simulink model "SF044A_HowDetn"  (R2013b)
settings: Solver=FixedStepDiscrete  SolverMode=SingleTasking  StartTime=0.0  StopTime=1  FixedStep=0.002  RelTol=1e-3
values from neighbouring files (symbols this model uses):
  ABSLTHIFRQTQHILIM_HWNWTMTR_F32 = DataDict.Constant    [SF044A_HowDetn_DataDict.m]
  ABSLTHIFRQTQLOLIM_HWNWTMTR_F32 = DataDict.Constant    [SF044A_HowDetn_DataDict.m]
  ARCHGLBPRM_2MILLISEC_SEC_F32 = DataDict.Constant    [SF044A_HowDetn_DataDict.m]
  HOWDETNESTIMNLIM_ULS_F32 = DataDict.Constant    [SF044A_HowDetn_DataDict.m]
  HOWDETNESTIMNTHD_ULS_F32 = DataDict.Constant    [SF044A_HowDetn_DataDict.m]
  HowDetnHiFrqGainY = DataDict.Calibration    [SF044A_HowDetn_DataDict.m]
  HowDetnMinVehSpd = DataDict.Calibration    [SF044A_HowDetn_DataDict.m]
  HowDetnPercOfPrevHowEstim = DataDict.Calibration    [SF044A_HowDetn_DataDict.m]
  HowDetnSlewRate = DataDict.Calibration    [SF044A_HowDetn_DataDict.m]
  HowDetnVehSpd = DataDict.Calibration    [SF044A_HowDetn_DataDict.m]
libraries: Fil x14, FloatToFixd x6, NxtrLim x5, FixdToFloat x3, BilnrIntrpnMplX x2, NxtrAbslt x2, simulink x2, LnrIntrpn x1, LnrIntrpnDyn x1
(part 1 of 2)
settings Model: Creator=xzqqlw  LastModifiedBy=XZB1DB
settings SolverCC: AutoInsertRateTranBlk=on  InsertRTBMode=Always
settings DataIOCC: LimitDataPoints=off  SaveFormat=Structure  ReturnWorkspaceOutputs=on
settings OptimizationCC: BlockReduction=off  InlineParams=on  ZeroExternalMemoryAtStartup=off  ZeroInternalMemoryAtStartup=off  OptimizeModelRefInitCode=on  LifeSpan=1
settings DebuggingCC: SignalInfNanChecking=error  SignalRangeChecking=warning  UnderspecifiedInitializationDetection=Simplified  SolverPrmCheckMsg=error  InheritedTsInSrcMsg=error  DiscreteInheritContinuousMsg=error  SingleTaskRateTransMsg=error  TasksWithSamePriorityMsg=error  SigSpecEnsureSampleTimeMsg=error  CheckMatrixSingularityMsg=error  ParameterUnderflowMsg=error  ParameterPrecisionLossMsg=error  ParameterTunabilityLossMsg=error  FixptConstUnderflowMsg=warning  FixptConstOverflowMsg=warning  VectorMatrixConversionMsg=error  SignalLabelMismatchMsg=error  UnconnectedInputMsg=error  UnconnectedOutputMsg=error  UnconnectedLineMsg=error  SFcnCompatibilityMsg=error  UniqueDataStoreMsg=warning  BusObjectLabelMismatch=error  RootOutportRequireBusObject=error  AssertControl=DisableAll  ModelReferenceIOMsg=error  ModelReferenceVersionMismatchMessage=warning  ModelReferenceIOMismatchMessage=error  ModelReferenceCSMismatchMessage=warning  ModelReferenceDataLoggingMessage=error  StateNameClashWarn=warning  StrictBusMsg=ErrorOnBusTreatedAsVector  NonBusSignalsTreatedAsBus=error  SFUnexpectedBacktrackingDiag=error  SFInvalidInputDataAccessInChartInitDiag=error  SFNoUnconditionalDefaultTransitionDiag=error  SFTransitionOutsideNaturalParentDiag=error  SFUnconditionalTransitionShadowingDiag=error  SFUndirectedBroadcastEventsDiag=error
settings ModelReferenceCC: ModelReferenceNumInstancesAllowed=Single
settings RTWCC: SystemTargetFile=autosar.tlc  GenCodeOnly=on  TemplateMakefile=ert_default_tmf  Description=AUTOSAR  GenerateReport=on  ProcessScript=autosar_make_rtw_hook  LaunchReport=on
settings CodeAppCC: GenerateComments=off  IgnoreCustomStorageClasses=off  CustomSymbolStrType=$N$R$M  CustomSymbolStrBlkIO=$N$M  SimulinkBlockComments=off
settings STFCustomTargetCC: ParMdlRefBuildCompliant=on  CompOptLevelCompliant=on  IncludeMdlTerminateFcn=off  CombineOutputUpdateFcns=on  SuppressErrorStatus=on  ERTFirstTimeCompliant=on  ERTCustomFileBanners=on  SupportNonFinite=off  SupportComplex=off  SupportContinuousTime=off  SupportNonInlinedSFcns=off  MATLABClassNameForMDSCustomization=Simulink.SoftwareTarget.ERTCustomization  AutosarCompliant=on  GRTInterface=off  SystemTargetFile=autosar.tlc
settings ERTTargetCC: CodeReplacementLibrary=ANSI_C  ConcurrentExecutionCompliant=off  IncludeMdlTerminateFcn=off  SuppressErrorStatus=on  SupportNonFinite=off  SupportComplex=off  ModelStepFunctionPrototypeControlCompliant=off  CPPClassGenCompliant=off  AutosarCompliant=on  InlinedParameterPlacement=NonHierarchical  ERTCustomFileTemplate=example_file_process.tlc  EnableUserReplacementTypes=on

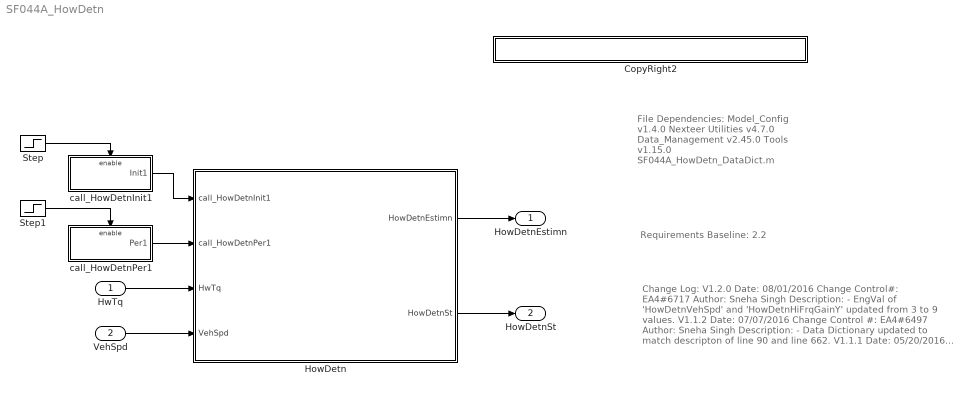
== system SF044A_HowDetn ==
  note: Change Log:
      |
      | V1.2.0
      | Date: 08/01/2016
      | Change Control#: EA4#6717
      | Author: Sneha Singh
      | Description:
      | - EngVal of 'HowDetnVehSpd' and 'HowDetnHiFrqGainY'
      | updated from 3 to 9 values.
      |
      | V1.1.2
      | Date: 07/07/2016
      | Change Control #: EA4#6497
      | Author: Sneha Singh
      | Description:
      | - Data Dictionary updated to match descripton
      | of line 90 and line 662.
      |
      | V1.1.1
      | Date: 05/20/2016
      | Change Control #: EA4#5844
      | Author: Sneha Singh
      | Description:
      | - Model traceability performed in DOORS.
      |
      | V 1.1.0
      | Date : 2/9/2016
      | Change Control #: EA4#2979
      | Author : Sudeep Shankar
      | Description:
      | - Limit block added to outputs 'HowDetnEstimn'.
      | and 'HowDetnSt'
      | - Updated DD to include 4 new constants
      |
      | V 1.0.0
      | Date: 1/14/2016
      | Change Control #: EA4#2979
      | Author: Sudeep Shankar
      | Description:
      | - Initial Release Based on EA3 V 1.0.0
  note: File Dependencies:
      |
      | Model_Config v1.4.0
      | Nexteer Utilities v4.7.0
      | Data_Management v2.45.0
      | Tools v1.15.0
      | SF044A_HowDetn_DataDict.m
  note: Requirements Baseline: 2.2
  HwTq : Inport  RequirementInfo={'linktype_rmi_doors' '0000baa4 (/E-STEER Core/SubSystem Specifications/Application Functions/SF044A HOW)' '#SF044A_67' 'true' 'REQ:SF044A_67' '' } %GIDa_72f413cc_dc3e_4eb0_8a2d_65e9c1fff85e
  VehSpd : Inport  RequirementInfo={'linktype_rmi_doors' '0000baa4 (/E-STEER Core/SubSystem Specifications/Application Functions/SF044A HOW)' '#SF044A_68' 'true' 'REQ:SF044A_68' '' } %GIDa_cc4347af_bdaf_4f30_b9d2_4f20a9b04acc  Port=2
  CopyRight2 : Subsystem  Description=|  mask(Copyright Information){none=on}
      | Copyright info block.                                               
      |                                                                     
      | Place copyright information at the top of every subsystem in design.
      mask prompts: none "No parameters"
      mask help: Place copyright information at the top of every subsystem in design.
      mask Display:
      | NxtrConf = 'Nexteer Confidential';
      | 
      | sys = bdroot; %handle for the current model ("system")
      | first = get_param(sys,'Created');
      | if(isempty(first))
      |     first = datestr(now,'yyyy');
      | else
      |     first = first(end-3:end);  %year is last four digits
      | end
      | 
      | last = get_param(sys,'LastModifiedDate');
      | if isempty(last)
      |     last = datestr(now,'yyyy');
      | else
      |     last = last(end-3:end);
      | end
      | 
      | if strcmp(first,last)
      |     fprintf('%s -- Copyright %s Nexteer',NxtrConf,first)
      | else
      |     fprintf('%s -- %s%s- %s Nexteer',NxtrConf,char(169),first,last)
      | end
  HowDetn : Subsystem
  Step : Step  Time=.001  Before=1  After=0  SampleTime=0
  Step1 : Step  Time=.001  SampleTime=0
  call_HowDetnInit1 : Subsystem  TreatAsAtomicUnit=on
  call_HowDetnPer1 : Subsystem  TreatAsAtomicUnit=on
  HowDetnEstimn : Outport  RequirementInfo={'linktype_rmi_doors' '0000baa4 (/E-STEER Core/SubSystem Specifications/Application Functions/SF044A HOW)' '#SF044A_69' 'true' 'REQ:SF044A_69' '' } %GIDa_72335151_86e3_4c12_b306_092b88286120
  HowDetnSt : Outport  RequirementInfo={'linktype_rmi_doors' '0000baa4 (/E-STEER Core/SubSystem Specifications/Application Functions/SF044A HOW)' '#SF044A_70' 'true' 'REQ:SF044A_70' '' } %GIDa_5536db44_27aa_4fe7_bd69_6a82a7bbddee  Port=2
  wires:
  HwTq/1 -> HowDetn/3(HwTq)
  HowDetn/1(HowDetnEstimn) -> HowDetnEstimn/1
  VehSpd/1 -> HowDetn/4(VehSpd)
  call_HowDetnPer1/1(Per1) -> HowDetn/2(call_HowDetnPer1)
  Step/1 -> call_HowDetnInit1/Enable
  call_HowDetnInit1/1(Init1) -> HowDetn/1(call_HowDetnInit1)
  Step1/1 -> call_HowDetnPer1/Enable
  HowDetn/2(HowDetnSt) -> HowDetnSt/1

== system SF044A_HowDetn/CopyRight2 ==

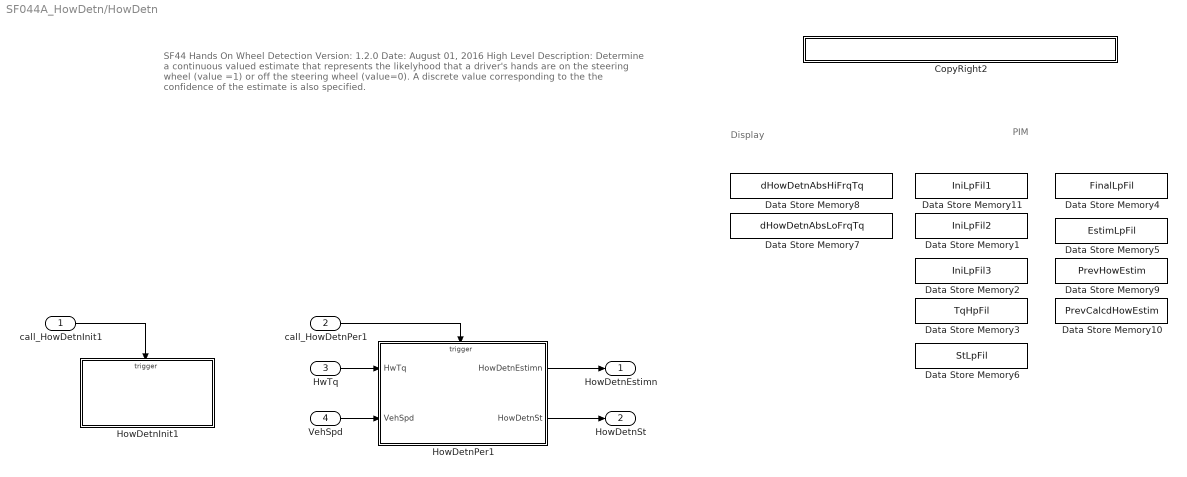
== system SF044A_HowDetn/HowDetn ==
  note: SF44 Hands On Wheel Detection
      |          Version:  1.2.0          Date: August 01, 2016
      |
      | High Level Description:
      | Determine a continuous valued estimate that represents the likelyhood that a driver's hands are
      | on the steering wheel (value =1) or off the steering wheel (value=0).  A discrete value corresponding
      | to the the confidence of the estimate is also specified.
  note: Display
  note: PIM
  call_HowDetnInit1 : Inport
  call_HowDetnPer1 : Inport  Port=2
  HwTq : Inport  Port=3
  VehSpd : Inport  Port=4
  CopyRight2 : Subsystem  Description=|  mask(Copyright Information){none=on}
      | Copyright info block.                                               
      |                                                                     
      | Place copyright information at the top of every subsystem in design.
      mask prompts: none "No parameters"
      mask help: Place copyright information at the top of every subsystem in design.
      mask Display:
      | NxtrConf = 'Nexteer Confidential';
      | 
      | sys = bdroot; %handle for the current model ("system")
      | first = get_param(sys,'Created');
      | first = first(end-3:end);  %year is last four digits
      | 
      | last = get_param(sys,'LastModifiedDate');
      | if isempty(last)
      |     last = datestr(now,'yyyy');
      | else
      |     last = last(end-3:end);
      | end
      | 
      | if strcmp(first,last)
      |     fprintf('%s -- Copyright %s Nexteer',NxtrConf,first)
      | else
      |     fprintf('%s -- %s%s- %s Nexteer',NxtrConf,char(169),first,last)
      | end
  Data Store Memory1 : DataStoreMemory  DataStoreName=IniLpFil2  InitialValue=struct( 'FilSt' , single(0) , 'FilGain', single(0) )  OutDataTypeStr=Bus: FilLpRec1  StateMustResolveToSignalObject=on
  Data Store Memory10 : DataStoreMemory  DataStoreName=PrevCalcdHowEstim  StateMustResolveToSignalObject=on
  Data Store Memory11 : DataStoreMemory  DataStoreName=IniLpFil1  InitialValue=struct( 'FilSt' , single(0) , 'FilGain', single(0) )  OutDataTypeStr=Bus: FilLpRec1  StateMustResolveToSignalObject=on
  Data Store Memory2 : DataStoreMemory  DataStoreName=IniLpFil3  InitialValue=struct( 'FilSt' , single(0) , 'FilGain', single(0) )  OutDataTypeStr=Bus: FilLpRec1  StateMustResolveToSignalObject=on
  Data Store Memory3 : DataStoreMemory  DataStoreName=TqHpFil  InitialValue=struct( 'FilLpRec' , struct( 'FilSt' , single(0) , 'FilGain', single(0) ) , 'CorrnFac', single(0) )  OutDataTypeStr=Bus: FilHpRec1  StateMustResolveToSignalObject=on
  Data Store Memory4 : DataStoreMemory  DataStoreName=FinalLpFil  InitialValue=struct( 'FilSt' , single(0) , 'FilGain', single(0) )  OutDataTypeStr=Bus: FilLpRec1  StateMustResolveToSignalObject=on
  Data Store Memory5 : DataStoreMemory  DataStoreName=EstimLpFil  InitialValue=struct( 'FilSt' , single(0) , 'FilGain', single(0) )  OutDataTypeStr=Bus: FilLpRec1  StateMustResolveToSignalObject=on
  Data Store Memory6 : DataStoreMemory  DataStoreName=StLpFil  InitialValue=[]  OutDataTypeStr=Bus: FilLpRec1  StateMustResolveToSignalObject=on
  Data Store Memory7 : DataStoreMemory  DataStoreName=dHowDetnAbsLoFrqTq  StateMustResolveToSignalObject=on
  Data Store Memory8 : DataStoreMemory  DataStoreName=dHowDetnAbsHiFrqTq  StateMustResolveToSignalObject=on
  Data Store Memory9 : DataStoreMemory  DataStoreName=PrevHowEstim  StateMustResolveToSignalObject=on
  HowDetnInit1 : Subsystem
  HowDetnPer1 : Subsystem  RequirementInfo={} %GIDa_2a73c725_3b58_4254_b96a_f86bf171ea48
  HowDetnEstimn : Outport
  HowDetnSt : Outport  Port=2
  wires:
  HwTq/1 -> HowDetnPer1/1(HwTq)
  call_HowDetnPer1/1 -> HowDetnPer1/Trigger
  call_HowDetnInit1/1 -> HowDetnInit1/Trigger
  HowDetnPer1/1(HowDetnEstimn) -> HowDetnEstimn/1
  HowDetnPer1/2(HowDetnSt) -> HowDetnSt/1
  VehSpd/1 -> HowDetnPer1/2(VehSpd)

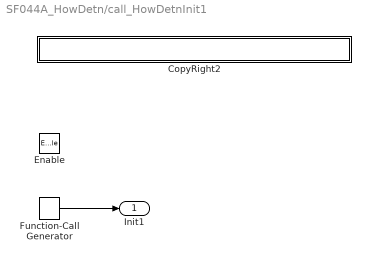
== system SF044A_HowDetn/call_HowDetnInit1 ==
  Enable : EnablePort
  CopyRight2 : Subsystem  Description=|  mask(Copyright Information){none=on}
      | Copyright info block.                                               
      |                                                                     
      | Place copyright information at the top of every subsystem in design.
      mask prompts: none "No parameters"
      mask help: Place copyright information at the top of every subsystem in design.
      mask Display:
      | NxtrConf = 'Nexteer Confidential';
      | 
      | sys = bdroot; %handle for the current model ("system")
      | first = get_param(sys,'Created');
      | if(isempty(first))
      |     first = datestr(now,'yyyy');
      | else
      |     first = first(end-3:end);  %year is last four digits
      | end
      | 
      | last = get_param(sys,'LastModifiedDate');
      | if isempty(last)
      |     last = datestr(now,'yyyy');
      | else
      |     last = last(end-3:end);
      | end
      | 
      | if strcmp(first,last)
      |     fprintf('%s -- Copyright %s Nexteer',NxtrConf,first)
      | else
      |     fprintf('%s -- %s%s- %s Nexteer',NxtrConf,char(169),first,last)
      | end
  Function-Call Generator : simulink/Ports & Subsystems/Function-Call Generator  sample_time=.004  numberOfIterations=1
  Init1 : Outport
  wires:
  Function-Call Generator/1 -> Init1/1

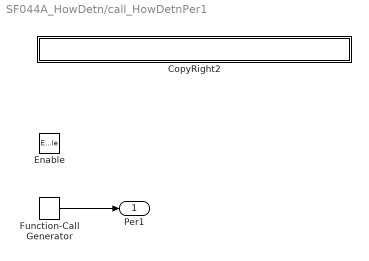
== system SF044A_HowDetn/call_HowDetnPer1 ==
  Enable : EnablePort
  CopyRight2 : Subsystem  Description=|  mask(Copyright Information){none=on}
      | Copyright info block.                                               
      |                                                                     
      | Place copyright information at the top of every subsystem in design.
      mask prompts: none "No parameters"
      mask help: Place copyright information at the top of every subsystem in design.
      mask Display:
      | NxtrConf = 'Nexteer Confidential';
      | 
      | sys = bdroot; %handle for the current model ("system")
      | first = get_param(sys,'Created');
      | if(isempty(first))
      |     first = datestr(now,'yyyy');
      | else
      |     first = first(end-3:end);  %year is last four digits
      | end
      | 
      | last = get_param(sys,'LastModifiedDate');
      | if isempty(last)
      |     last = datestr(now,'yyyy');
      | else
      |     last = last(end-3:end);
      | end
      | 
      | if strcmp(first,last)
      |     fprintf('%s -- Copyright %s Nexteer',NxtrConf,first)
      | else
      |     fprintf('%s -- %s%s- %s Nexteer',NxtrConf,char(169),first,last)
      | end
  Function-Call Generator : simulink/Ports & Subsystems/Function-Call Generator  sample_time=.004  numberOfIterations=1
  Per1 : Outport
  wires:
  Function-Call Generator/1 -> Per1/1

== system SF044A_HowDetn/HowDetn/CopyRight2 ==

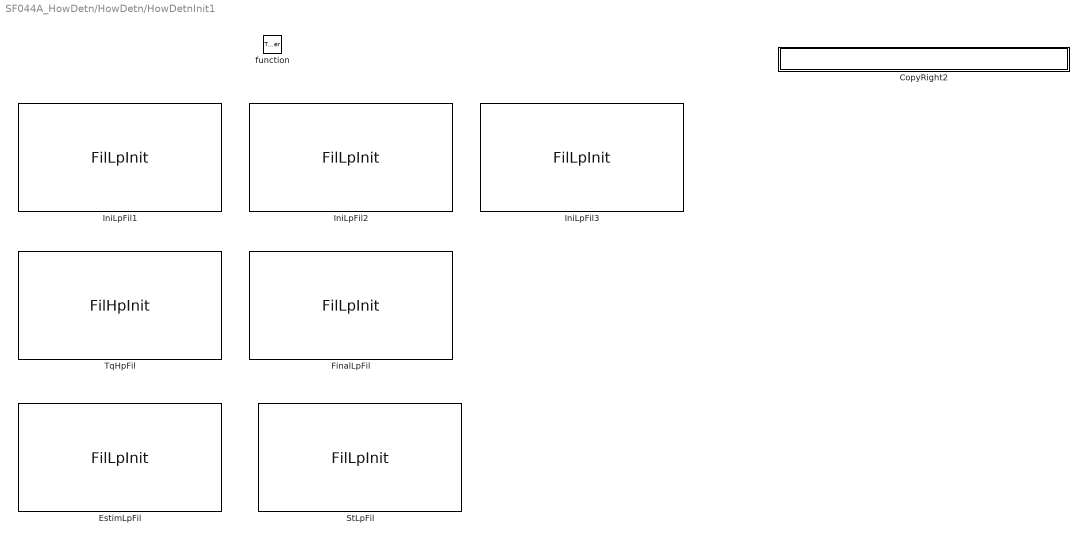
== system SF044A_HowDetn/HowDetn/HowDetnInit1 ==
  function : TriggerPort  TriggerType=function-call
  CopyRight2 : Subsystem  Description=|  mask(Copyright Information){none=on}
      | Copyright info block.                                               
      |                                                                     
      | Place copyright information at the top of every subsystem in design.
      mask prompts: none "No parameters"
      mask help: Place copyright information at the top of every subsystem in design.
      mask Display:
      | NxtrConf = 'Nexteer Confidential';
      | 
      | sys = bdroot; %handle for the current model ("system")
      | first = get_param(sys,'Created');
      | if(isempty(first))
      |     first = datestr(now,'yyyy');
      | else
      |     first = first(end-3:end);  %year is last four digits
      | end
      | 
      | last = get_param(sys,'LastModifiedDate');
      | if isempty(last)
      |     last = datestr(now,'yyyy');
      | else
      |     last = last(end-3:end);
      | end
      | 
      | if strcmp(first,last)
      |     fprintf('%s -- Copyright %s Nexteer',NxtrConf,first)
      | else
      |     fprintf('%s -- %s%s- %s Nexteer',NxtrConf,char(169),first,last)
      | end
  EstimLpFil : Fil/FilLpInit  Ic=0  Ts=ARCHGLBPRM_2MILLISEC_SEC_F32  Freq=HowDetnEstimLpFilFrq  StVar=EstimLpFil
  FinalLpFil : Fil/FilLpInit  Ic=0  Ts=ARCHGLBPRM_2MILLISEC_SEC_F32  Freq=HowDetnTqFinalLpFilFrq  StVar=FinalLpFil
  IniLpFil1 : Fil/FilLpInit  Ic=0  Ts=ARCHGLBPRM_2MILLISEC_SEC_F32  Freq=HowDetnTqInitLpFilFrq  StVar=IniLpFil1
  IniLpFil2 : Fil/FilLpInit  Ic=0  Ts=ARCHGLBPRM_2MILLISEC_SEC_F32  Freq=HowDetnTqInitLpFilFrq  StVar=IniLpFil2
  IniLpFil3 : Fil/FilLpInit  Ic=0  Ts=ARCHGLBPRM_2MILLISEC_SEC_F32  Freq=HowDetnTqInitLpFilFrq  StVar=IniLpFil3
  StLpFil : Fil/FilLpInit  Ic=0  Ts=ARCHGLBPRM_2MILLISEC_SEC_F32  Freq=HowDetnStLpFilFrq  StVar=StLpFil
  TqHpFil : Fil/FilHpInit  Ic=0  Ts=ARCHGLBPRM_2MILLISEC_SEC_F32  Freq=HowDetnTqHpFilFrq  StVar=TqHpFil
      link override FilHpUpdGain/FilLpUpdGain/Data Store Write: DataStoreName=TqHpFil  DataStoreElements=TqHpFil.FilLpRec.FilGain

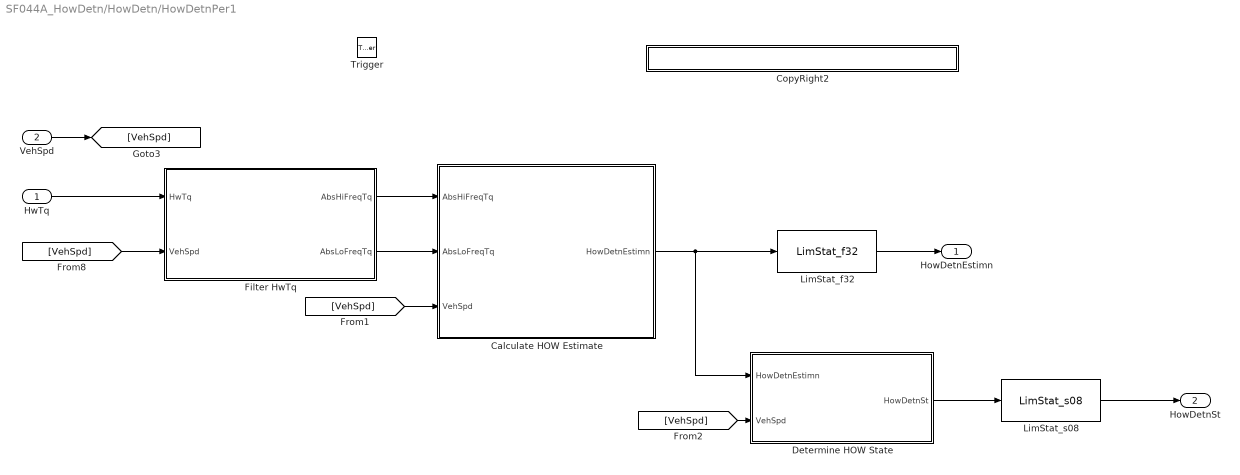
== system SF044A_HowDetn/HowDetn/HowDetnPer1 ==
  HwTq : Inport
  VehSpd : Inport  Port=2
  Trigger : TriggerPort  TriggerType=function-call  PortDimensions=1
  Calculate HOW Estimate : Subsystem  RequirementInfo={} %GIDa_125b53e8_c1e4_47fd_8eb9_c9154c9b4f28
  CopyRight2 : Subsystem  Description=|  mask(Copyright Information){none=on}
      | Copyright info block.                                               
      |                                                                     
      | Place copyright information at the top of every subsystem in design.
      mask prompts: none "No parameters"
      mask help: Place copyright information at the top of every subsystem in design.
      mask Display:
      | NxtrConf = 'Nexteer Confidential';
      | 
      | sys = bdroot; %handle for the current model ("system")
      | first = get_param(sys,'Created');
      | first = first(end-3:end);  %year is last four digits
      | 
      | last = get_param(sys,'LastModifiedDate');
      | if isempty(last)
      |     last = datestr(now,'yyyy');
      | else
      |     last = last(end-3:end);
      | end
      | 
      | if strcmp(first,last)
      |     fprintf('%s -- Copyright %s Nexteer',NxtrConf,first)
      | else
      |     fprintf('%s -- %s%s- %s Nexteer',NxtrConf,char(169),first,last)
      | end
  Determine HOW State : Subsystem
  Filter HwTq : Subsystem
  LimStat_f32 : NxtrLim/LimStat_f32  RequirementInfo={'linktype_rmi_doors' '0000baa4 (/E-STEER Core/SubSystem Specifications/Application Functions/SF044A HOW)' '#SF044A_86' 'true' 'REQ:SF044A_86' '' } %GIDa_8c16cf74_aa0f_484a_aba3_a9bc207344b8  LoLim=HOWDETNESTIMNLOLIM_ULS_F32  HiLim=HOWDETNESTIMNHILIM_ULS_F32
      settings: AttributesFormatString=|
      | Low Limit: %<LoLim>
      | High Limit:%<HiLim>
  LimStat_s08 : NxtrLim/LimStat_s08  RequirementInfo={'linktype_rmi_doors' '0000baa4 (/E-STEER Core/SubSystem Specifications/Application Functions/SF044A HOW)' '#SF044A_87' 'true' 'REQ:SF044A_87' '' } %GIDa_b47c45be_9a65_48c3_bad3_da8eb273219c  LoLim=HOWDETNSTLOLIM_CNT_S08  HiLim=HOWDETNSTHILIM_CNT_S08
      settings: AttributesFormatString=|
      | Low Limit: %<LoLim>
      | High Limit:%<HiLim>
  HowDetnEstimn : Outport
  HowDetnSt : Outport  Port=2
  wires:
  Filter HwTq/2(AbsLoFreqTq) -> Calculate HOW Estimate/2(AbsLoFreqTq)
  Filter HwTq/1(AbsHiFreqTq) -> Calculate HOW Estimate/1(AbsHiFreqTq)
  HwTq/1 -> Filter HwTq/1(HwTq)
  VehSpd/1 -> [VehSpd]
  [VehSpd] -> Filter HwTq/2(VehSpd)
  [VehSpd] -> Calculate HOW Estimate/3(VehSpd)
  Determine HOW State/1(HowDetnSt) -> LimStat_s08/1
  Calculate HOW Estimate/1(HowDetnEstimn) -> LimStat_f32/1, Determine HOW State/1(HowDetnEstimn)
  [VehSpd] -> Determine HOW State/2(VehSpd)
  LimStat_f32/1 -> HowDetnEstimn/1
  LimStat_s08/1 -> HowDetnSt/1

== system SF044A_HowDetn/call_HowDetnInit1/CopyRight2 ==

== system SF044A_HowDetn/call_HowDetnPer1/CopyRight2 ==

== system SF044A_HowDetn/HowDetn/HowDetnInit1/CopyRight2 ==

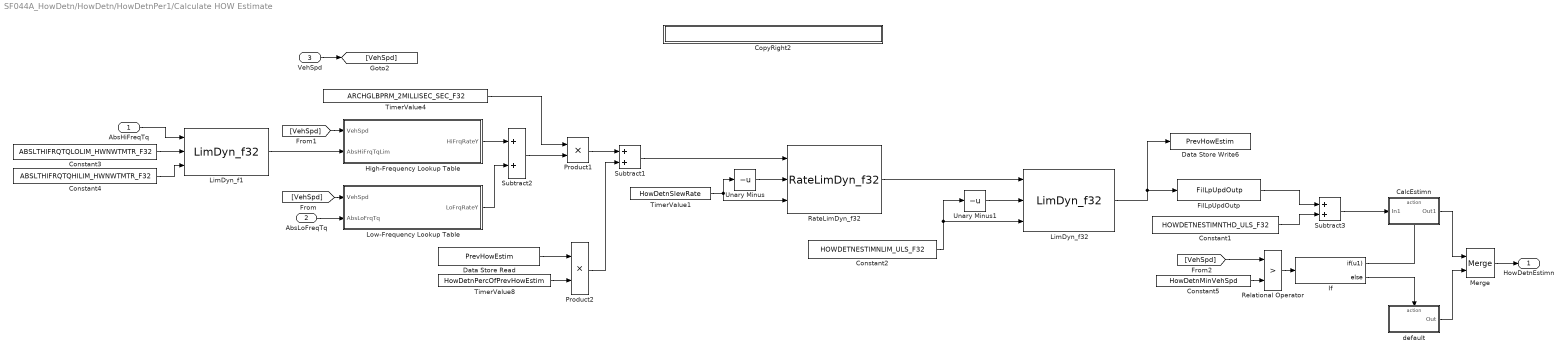
== system SF044A_HowDetn/HowDetn/HowDetnPer1/Calculate HOW Estimate ==
  AbsHiFreqTq : Inport
  AbsLoFreqTq : Inport  Port=2
  VehSpd : Inport  Port=3
  CalcEstimn : Subsystem  RequirementInfo={} %GIDa_617fa122_fba1_40f3_ae82_fa9f065f1001  TreatAsAtomicUnit=on
  Constant1 : Constant  RequirementInfo={'linktype_rmi_doors' '0000baa4 (/E-STEER Core/SubSystem Specifications/Application Functions/SF044A HOW)' '#SF044A_9' 'true' 'REQ:SF044A_9' '' } %GIDa_510134ec_df2a_44f3_b6a7_445b19eb384f  Value=HOWDETNESTIMNTHD_ULS_F32  OutDataTypeStr=single
  Constant2 : Constant  RequirementInfo={'linktype_rmi_doors' '0000baa4 (/E-STEER Core/SubSystem Specifications/Application Functions/SF044A HOW)' '#SF044A_9' 'true' 'REQ:SF044A_9' '' } %GIDa_5dfda7fa_5804_4bb8_aabe_6e7cbeab5332  Value=HOWDETNESTIMNLIM_ULS_F32  OutDataTypeStr=single
  Constant3 : Constant  Value=ABSLTHIFRQTQLOLIM_HWNWTMTR_F32  OutDataTypeStr=single
  Constant4 : Constant  Value=ABSLTHIFRQTQHILIM_HWNWTMTR_F32  OutDataTypeStr=single
  Constant5 : Constant  RequirementInfo={'linktype_rmi_doors' '0000baa4 (/E-STEER Core/SubSystem Specifications/Application Functions/SF044A HOW)' '#SF044A_11' 'true' 'REQ:SF044A_11' '' } %GIDa_59fd2d45_5b8c_4efd_b03d_e76d89bd0eb2  Value=HowDetnMinVehSpd
  CopyRight2 : Subsystem  Description=|  mask(Copyright Information){none=on}
      | Copyright info block.                                               
      |                                                                     
      | Place copyright information at the top of every subsystem in design.
      mask prompts: none "No parameters"
      mask help: Place copyright information at the top of every subsystem in design.
      mask Display:
      | NxtrConf = 'Nexteer Confidential';
      | 
      | sys = bdroot; %handle for the current model ("system")
      | first = get_param(sys,'Created');
      | first = first(end-3:end);  %year is last four digits
      | 
      | last = get_param(sys,'LastModifiedDate');
      | if isempty(last)
      |     last = datestr(now,'yyyy');
      | else
      |     last = last(end-3:end);
      | end
      | 
      | if strcmp(first,last)
      |     fprintf('%s -- Copyright %s Nexteer',NxtrConf,first)
      | else
      |     fprintf('%s -- %s%s- %s Nexteer',NxtrConf,char(169),first,last)
      | end
  Data Store Read : DataStoreRead  DataStoreName=PrevHowEstim
  Data Store Write6 : DataStoreWrite  DataStoreName=PrevHowEstim
  FilLpUpdOutp : Fil/FilLpUpdOutp  RequirementInfo={'linktype_rmi_doors' '0000baa4 (/E-STEER Core/SubSystem Specifications/Application Functions/SF044A HOW)' '#SF044A_9' 'true' 'REQ:SF044A_9' '' } %GIDa_2bf98463_0e11_4c11_baa4_3d7784cd32c8  StVar=EstimLpFil
      settings: AttributesFormatString=StVar: %<StVar>
  High-Frequency Lookup Table : Subsystem  RequirementInfo={} %GIDa_275c464c_37aa_4e65_a316_f717549d41e8
  If : If  RequirementInfo={'linktype_rmi_doors' '0000baa4 (/E-STEER Core/SubSystem Specifications/Application Functions/SF044A HOW)' '#SF044A_11' 'true' 'REQ:SF044A_11' '' } %GIDa_9873cb79_688d_4723_9a75_1f2f6a65a748  IfExpression=u1
  LimDyn_f1 : NxtrLim/LimDyn_f32
  LimDyn_f32 : NxtrLim/LimDyn_f32  RequirementInfo={'linktype_rmi_doors' '0000baa4 (/E-STEER Core/SubSystem Specifications/Application Functions/SF044A HOW)' '#SF044A_9' 'true' 'REQ:SF044A_9' '' } %GIDa_afc9474c_9e21_4218_8860_b1c19bd74f60
  Low-Frequency Lookup Table : Subsystem  RequirementInfo={} %GIDa_9e3951b9_ca3e_4007_b783_1f414f53d997
  Merge : Merge  RequirementInfo={} %GIDa_e828a7f0_5398_48af_90ba_2c23b3566db0
  Product1 : Product  SaturateOnIntegerOverflow=on  OutDataTypeStr=Inherit: Same as first input
  Product2 : Product  SaturateOnIntegerOverflow=on  OutDataTypeStr=Inherit: Same as first input
  RateLimDyn_f32 : NxtrLim/RateLimDyn_f32  StVar=PrevCalcdHowEstim  Ts=ARCHGLBPRM_2MILLISEC_SEC_F32
      settings: AttributesFormatString=StVar: %<StVar>
  Relational Operator : RelationalOperator  RequirementInfo={'linktype_rmi_doors' '0000baa4 (/E-STEER Core/SubSystem Specifications/Application Functions/SF044A HOW)' '#SF044A_11' 'true' 'REQ:SF044A_11' '' } %GIDa_168d8172_153e_44a6_b364_010bf1f47def  Operator=>  OutDataTypeStr=boolean
  Subtract1 : Sum
  Subtract2 : Sum
  Subtract3 : Sum  RequirementInfo={'linktype_rmi_doors' '0000baa4 (/E-STEER Core/SubSystem Specifications/Application Functions/SF044A HOW)' '#SF044A_9' 'true' 'REQ:SF044A_9' '' } %GIDa_2d4330ff_3f14_4946_8c72_82438943e93e
  TimerValue1 : Constant  RequirementInfo={'linktype_rmi_doors' '0000baa4 (/E-STEER Core/SubSystem Specifications/Application Functions/SF044A HOW)' '#SF044A_21' 'true' 'REQ:SF044A_21' '' } %GIDa_04706bfd_cd74_4c86_9394_ff4021b4c8a7  Value=HowDetnSlewRate
  TimerValue4 : Constant  Value=ARCHGLBPRM_2MILLISEC_SEC_F32
  TimerValue8 : Constant  Value=HowDetnPercOfPrevHowEstim
  Unary Minus : UnaryMinus
  Unary Minus1 : UnaryMinus  RequirementInfo={'linktype_rmi_doors' '0000baa4 (/E-STEER Core/SubSystem Specifications/Application Functions/SF044A HOW)' '#SF044A_9' 'true' 'REQ:SF044A_9' '' } %GIDa_312a9058_0735_44ac_8fa7_5a3b33df9045
  default : Subsystem  RequirementInfo={'linktype_rmi_doors' '0000baa4 (/E-STEER Core/SubSystem Specifications/Application Functions/SF044A HOW)' '#SF044A_11' 'true' 'REQ:SF044A_11' '' ; 'linktype_rmi_doors' '0000baa4 (/E-STEER Core/SubSystem Specifications/Application Functions/SF044A HOW)' '#SF044A_10' 'true' 'REQ:SF044A_10' '' } %GIDa_ce223202_4df6_49c5_af8b_b99d8f0294fd  TreatAsAtomicUnit=on
  HowDetnEstimn : Outport  RequirementInfo={'linktype_rmi_doors' '0000baa4 (/E-STEER Core/SubSystem Specifications/Application Functions/SF044A HOW)' '#SF044A_83' 'true' 'REQ:SF044A_83' '' } %GIDa_ef1fc6b4_f2c6_4ead_beb3_33b8d5da1105
  wires:
  [VehSpd] -> Low-Frequency Lookup Table/1(VehSpd)
  TimerValue4/1 -> Product1/1
  [VehSpd] -> High-Frequency Lookup Table/1(VehSpd)
  TimerValue8/1 -> Product2/2
  Product2/1 -> Subtract1/2
  LimDyn_f32/1 -> Data Store Write6/1, FilLpUpdOutp/1
  Constant1/1 -> Subtract3/2
  Relational Operator/1 -> If/1
  [VehSpd] -> Relational Operator/1
  Low-Frequency Lookup Table/1(LoFrqRateY) -> Subtract2/2
  High-Frequency Lookup Table/1(HiFrqRateY) -> Subtract2/1
  VehSpd/1 -> [VehSpd]
  AbsLoFreqTq/1 -> Low-Frequency Lookup Table/2(AbsLoFrqTq)
  AbsHiFreqTq/1 -> LimDyn_f1/1
  Product1/1 -> Subtract1/1
  Subtract1/1 -> RateLimDyn_f32/1
  Subtract2/1 -> Product1/2
  Merge/1 -> HowDetnEstimn/1
  FilLpUpdOutp/1 -> Subtract3/1
  Subtract3/1 -> CalcEstimn/1(In1)
  LimDyn_f1/1 -> High-Frequency Lookup Table/2(AbsHiFrqTqLim)
  Data Store Read/1 -> Product2/1
  TimerValue1/1 -> Unary Minus/1, RateLimDyn_f32/3
  Unary Minus/1 -> RateLimDyn_f32/2
  RateLimDyn_f32/1 -> LimDyn_f32/1
  Constant2/1 -> LimDyn_f32/3, Unary Minus1/1
  Unary Minus1/1 -> LimDyn_f32/2
  Constant3/1 -> LimDyn_f1/2
  Constant4/1 -> LimDyn_f1/3
  Constant5/1 -> Relational Operator/2
  If/1 -> CalcEstimn/Action
  If/2 -> default/Action
  CalcEstimn/1(Out1) -> Merge/1
  default/1(Out) -> Merge/2

== system SF044A_HowDetn/HowDetn/HowDetnPer1/CopyRight2 ==

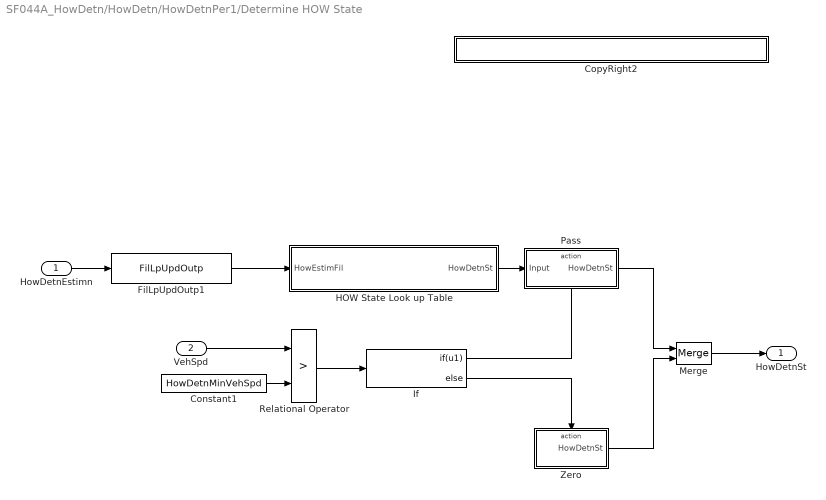
== system SF044A_HowDetn/HowDetn/HowDetnPer1/Determine HOW State ==
  HowDetnEstimn : Inport  RequirementInfo={'linktype_rmi_doors' '0000baa4 (/E-STEER Core/SubSystem Specifications/Application Functions/SF044A HOW)' '#SF044A_22' 'true' 'REQ:SF044A_22' '' } %GIDa_03cf274d_e1d4_4735_9e68_3ddfe4e3cced
  VehSpd : Inport  RequirementInfo={'linktype_rmi_doors' '0000baa4 (/E-STEER Core/SubSystem Specifications/Application Functions/SF044A HOW)' '#SF044A_15' 'true' 'REQ:SF044A_15' '' } %GIDa_07049647_5da3_4b2f_a8e0_024028ea6550  Port=2
  Constant1 : Constant  RequirementInfo={'linktype_rmi_doors' '0000baa4 (/E-STEER Core/SubSystem Specifications/Application Functions/SF044A HOW)' '#SF044A_15' 'true' 'REQ:SF044A_15' '' } %GIDa_c179c529_5319_48e2_b362_6271d68d3d51  Value=HowDetnMinVehSpd
  CopyRight2 : Subsystem  Description=|  mask(Copyright Information){none=on}
      | Copyright info block.                                               
      |                                                                     
      | Place copyright information at the top of every subsystem in design.
      mask prompts: none "No parameters"
      mask help: Place copyright information at the top of every subsystem in design.
      mask Display:
      | NxtrConf = 'Nexteer Confidential';
      | 
      | sys = bdroot; %handle for the current model ("system")
      | first = get_param(sys,'Created');
      | first = first(end-3:end);  %year is last four digits
      | 
      | last = get_param(sys,'LastModifiedDate');
      | if isempty(last)
      |     last = datestr(now,'yyyy');
      | else
      |     last = last(end-3:end);
      | end
      | 
      | if strcmp(first,last)
      |     fprintf('%s -- Copyright %s Nexteer',NxtrConf,first)
      | else
      |     fprintf('%s -- %s%s- %s Nexteer',NxtrConf,char(169),first,last)
      | end
  FilLpUpdOutp1 : Fil/FilLpUpdOutp  RequirementInfo={'linktype_rmi_doors' '0000baa4 (/E-STEER Core/SubSystem Specifications/Application Functions/SF044A HOW)' '#SF044A_22' 'true' 'REQ:SF044A_22' '' } %GIDa_4d5be9a8_a45d_476e_ab1c_4985aa05426d  StVar=StLpFil
      settings: AttributesFormatString=StVar: %<StVar>
  HOW State Look up Table : Subsystem  RequirementInfo={'linktype_rmi_doors' '0000baa4 (/E-STEER Core/SubSystem Specifications/Application Functions/SF044A HOW)' '#SF044A_13' 'true' 'REQ:SF044A_13' '' ; 'linktype_rmi_doors' '0000baa4 (/E-STEER Core/SubSystem Specifications/Application Functions/SF044A HOW)' '#SF044A_16' 'true' 'REQ:SF044A_16' '' ; 'linktype_rmi_doors' '0000baa4 (/E-STEER Core/SubSystem Specifications/Application Functions/SF044A HOW)' '#SF044A_17' 'true' 'REQ:SF044A_17' '' ; 'linktype_rmi_doors' '0000baa4 (/E-STEER Core/SubSystem Specifications/Application Functions/SF044A HOW)' '#SF044A_18' 'true' 'REQ:SF044A_18' '' ; 'linktype_rmi_doors' '0000baa4 (/E-STEER Core/SubSystem Specifications/Application Functions/SF044A HOW)' '#SF044A_19' 'true' 'REQ:SF044A_19' '' ; 'linktype_rmi_doors' '0000baa4 (/E-STEER Core/SubSystem Specifications/Application Functions/SF044A HOW)' '#SF044A_22' 'true' 'REQ:SF044A_22' '' } %GIDa_438012bb_0bfc_4c7b_af61_70c74288710f
  If : If  RequirementInfo={'linktype_rmi_doors' '0000baa4 (/E-STEER Core/SubSystem Specifications/Application Functions/SF044A HOW)' '#SF044A_15' 'true' 'REQ:SF044A_15' '' } %GIDa_0a225032_c3f6_4d32_8981_c29469b8ba46  IfExpression=u1
  Merge : Merge
  Pass : Subsystem  RequirementInfo={} %GIDa_13f45ff3_ba3e_4861_a525_81327e2c7efe  TreatAsAtomicUnit=on
  Relational Operator : RelationalOperator  RequirementInfo={'linktype_rmi_doors' '0000baa4 (/E-STEER Core/SubSystem Specifications/Application Functions/SF044A HOW)' '#SF044A_15' 'true' 'REQ:SF044A_15' '' } %GIDa_4fb3389c_a442_41f6_a4ae_ec136e4d3385  Operator=>  OutDataTypeStr=boolean
  Zero : Subsystem  RequirementInfo={'linktype_rmi_doors' '0000baa4 (/E-STEER Core/SubSystem Specifications/Application Functions/SF044A HOW)' '#SF044A_14' 'true' 'REQ:SF044A_14' '' ; 'linktype_rmi_doors' '0000baa4 (/E-STEER Core/SubSystem Specifications/Application Functions/SF044A HOW)' '#SF044A_15' 'true' 'REQ:SF044A_15' '' } %GIDa_15ffa420_2f46_451d_a55c_dc4254f46d2e  TreatAsAtomicUnit=on
  HowDetnSt : Outport  RequirementInfo={'linktype_rmi_doors' '0000baa4 (/E-STEER Core/SubSystem Specifications/Application Functions/SF044A HOW)' '#SF044A_12' 'true' 'REQ:SF044A_12' '' } %GIDa_f85ec72f_3c46_4aec_be62_6aba09814511
  wires:
  HOW State Look up Table/1(HowDetnSt) -> Pass/1(Input)
  HowDetnEstimn/1 -> FilLpUpdOutp1/1
  FilLpUpdOutp1/1 -> HOW State Look up Table/1(HowEstimFil)
  Relational Operator/1 -> If/1
  VehSpd/1 -> Relational Operator/1
  Constant1/1 -> Relational Operator/2
  If/2 -> Zero/Action
  Zero/1(HowDetnSt) -> Merge/2
  If/1 -> Pass/Action
  Pass/1(HowDetnSt) -> Merge/1
  Merge/1 -> HowDetnSt/1

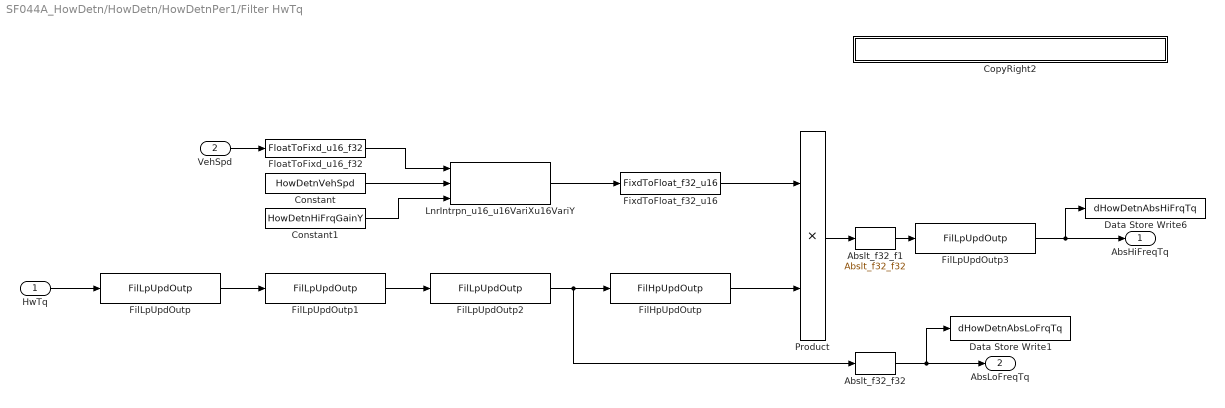
== system SF044A_HowDetn/HowDetn/HowDetnPer1/Filter HwTq ==
  HwTq : Inport  RequirementInfo={'linktype_rmi_doors' '0000baa4 (/E-STEER Core/SubSystem Specifications/Application Functions/SF044A HOW)' '#SF044A_80' 'true' 'REQ:SF044A_80' '' } %GIDa_cd4e38a2_3a6c_4305_9e2f_33452131362b
  VehSpd : Inport  RequirementInfo={'linktype_rmi_doors' '0000baa4 (/E-STEER Core/SubSystem Specifications/Application Functions/SF044A HOW)' '#SF044A_82' 'true' 'REQ:SF044A_82' '' } %GIDa_c953dac0_c289_4f03_82ce_9b6616f65fc0  Port=2
  Abslt_f32_f1 : NxtrAbslt/Abslt_f32_f32  RequirementInfo={'linktype_rmi_doors' '0000baa4 (/E-STEER Core/SubSystem Specifications/Application Functions/SF044A HOW)' '#SF044A_82' 'true' 'REQ:SF044A_82' '' } %GIDa_e092a889_5582_43d8_8ee9_d8cfed7db834  SFunctionSpec=single y1 = Abslt_f32_f32(single u1)
      settings: AttributesFormatString=%<Name>
  Abslt_f32_f32 : NxtrAbslt/Abslt_f32_f32  RequirementInfo={'linktype_rmi_doors' '0000baa4 (/E-STEER Core/SubSystem Specifications/Application Functions/SF044A HOW)' '#SF044A_80' 'true' 'REQ:SF044A_80' '' } %GIDa_75bc82c3_f017_4405_8b5d_e0bad32f3326  SFunctionSpec=single y1 = Abslt_f32_f32(single u1)
      settings: AttributesFormatString=%<Name>
  Constant : Constant  RequirementInfo={'linktype_rmi_doors' '0000baa4 (/E-STEER Core/SubSystem Specifications/Application Functions/SF044A HOW)' '#SF044A_82' 'true' 'REQ:SF044A_82' '' } %GIDa_c1668684_a190_4162_a3bf_3d4511b721a0  Value=HowDetnVehSpd
  Constant1 : Constant  RequirementInfo={'linktype_rmi_doors' '0000baa4 (/E-STEER Core/SubSystem Specifications/Application Functions/SF044A HOW)' '#SF044A_82' 'true' 'REQ:SF044A_82' '' } %GIDa_0cdb3428_a7ff_4fb4_b5fa_64baccde16a9  Value=HowDetnHiFrqGainY
  CopyRight2 : Subsystem  Description=|  mask(Copyright Information){none=on}
      | Copyright info block.                                               
      |                                                                     
      | Place copyright information at the top of every subsystem in design.
      mask prompts: none "No parameters"
      mask help: Place copyright information at the top of every subsystem in design.
      mask Display:
      | NxtrConf = 'Nexteer Confidential';
      | 
      | sys = bdroot; %handle for the current model ("system")
      | first = get_param(sys,'Created');
      | first = first(end-3:end);  %year is last four digits
      | 
      | last = get_param(sys,'LastModifiedDate');
      | if isempty(last)
      |     last = datestr(now,'yyyy');
      | else
      |     last = last(end-3:end);
      | end
      | 
      | if strcmp(first,last)
      |     fprintf('%s -- Copyright %s Nexteer',NxtrConf,first)
      | else
      |     fprintf('%s -- %s%s- %s Nexteer',NxtrConf,char(169),first,last)
      | end
  Data Store Write1 : DataStoreWrite  RequirementInfo={'linktype_rmi_doors' '0000baa4 (/E-STEER Core/SubSystem Specifications/Application Functions/SF044A HOW)' '#SF044A_80' 'true' 'REQ:SF044A_80' '' } %GIDa_89d069f4_be19_4fec_b4fb_2b35685090a3  DataStoreName=dHowDetnAbsLoFrqTq
  Data Store Write6 : DataStoreWrite  RequirementInfo={'linktype_rmi_doors' '0000baa4 (/E-STEER Core/SubSystem Specifications/Application Functions/SF044A HOW)' '#SF044A_82' 'true' 'REQ:SF044A_82' '' } %GIDa_b9df3445_512e_4094_9608_6372e97ea29d  DataStoreName=dHowDetnAbsHiFrqTq
  FilHpUpdOutp : Fil/FilHpUpdOutp  RequirementInfo={'linktype_rmi_doors' '0000baa4 (/E-STEER Core/SubSystem Specifications/Application Functions/SF044A HOW)' '#SF044A_81' 'true' 'REQ:SF044A_81' '' } %GIDa_1c9c8565_191c_4ea1_9db8_9014687bab3b  StVar=TqHpFil
      link override FilLpUpdOutp/Data Store Read: DataStoreName=TqHpFil  DataStoreElements=TqHpFil.FilLpRec.FilSt#TqHpFil.FilLpRec.FilGain
      settings: AttributesFormatString=StVar: %<StVar>
  FilLpUpdOutp : Fil/FilLpUpdOutp  RequirementInfo={'linktype_rmi_doors' '0000baa4 (/E-STEER Core/SubSystem Specifications/Application Functions/SF044A HOW)' '#SF044A_80' 'true' 'REQ:SF044A_80' '' } %GIDa_a5d3a247_379d_46c5_aa7e_bf548ab1f908  StVar=IniLpFil1
      settings: AttributesFormatString=StVar: %<StVar>
  FilLpUpdOutp1 : Fil/FilLpUpdOutp  RequirementInfo={'linktype_rmi_doors' '0000baa4 (/E-STEER Core/SubSystem Specifications/Application Functions/SF044A HOW)' '#SF044A_80' 'true' 'REQ:SF044A_80' '' } %GIDa_15cfc8f7_74dd_4908_9ab1_6aa981ba1881  StVar=IniLpFil2
      settings: AttributesFormatString=StVar: %<StVar>
  FilLpUpdOutp2 : Fil/FilLpUpdOutp  RequirementInfo={'linktype_rmi_doors' '0000baa4 (/E-STEER Core/SubSystem Specifications/Application Functions/SF044A HOW)' '#SF044A_80' 'true' 'REQ:SF044A_80' '' } %GIDa_2008d412_0440_4381_aa7f_d96427028035  StVar=IniLpFil3
      settings: AttributesFormatString=StVar: %<StVar>
  FilLpUpdOutp3 : Fil/FilLpUpdOutp  RequirementInfo={'linktype_rmi_doors' '0000baa4 (/E-STEER Core/SubSystem Specifications/Application Functions/SF044A HOW)' '#SF044A_82' 'true' 'REQ:SF044A_82' '' } %GIDa_d3a48c91_6f86_4eac_9e77_16bc55103697  StVar=FinalLpFil
      settings: AttributesFormatString=StVar: %<StVar>
  FixdToFloat_f32_u16 : FixdToFloat/FixdToFloat_f32_u16  RequirementInfo={'linktype_rmi_doors' '0000baa4 (/E-STEER Core/SubSystem Specifications/Application Functions/SF044A HOW)' '#SF044A_82' 'true' 'REQ:SF044A_82' '' } %GIDa_2d49d4ff_542e_49f7_b2c3_0da78f00f2a6  Param1=7
  FloatToFixd_u16_f32 : FloatToFixd/FloatToFixd_u16_f32  RequirementInfo={'linktype_rmi_doors' '0000baa4 (/E-STEER Core/SubSystem Specifications/Application Functions/SF044A HOW)' '#SF044A_82' 'true' 'REQ:SF044A_82' '' } %GIDa_e7f52add_40ff_4222_a128_7ffd3761c852  Param1=7
  LnrIntrpn_u16_u16VariXu16VariY : LnrIntrpnDyn/LnrIntrpn_u16_u16VariXu16VariY  RequirementInfo={'linktype_rmi_doors' '0000baa4 (/E-STEER Core/SubSystem Specifications/Application Functions/SF044A HOW)' '#SF044A_82' 'true' 'REQ:SF044A_82' '' } %GIDa_64fd5925_4f50_4fa2_b6ac_ceeb720e91db
      settings: AttributesFormatString=Lnr ( u16VariX , u16VariY )
  Product : Product  RequirementInfo={'linktype_rmi_doors' '0000baa4 (/E-STEER Core/SubSystem Specifications/Application Functions/SF044A HOW)' '#SF044A_82' 'true' 'REQ:SF044A_82' '' } %GIDa_4907a559_98c6_4c39_a1a7_7aef6e6490c4  RndMeth=Zero
  AbsHiFreqTq : Outport  RequirementInfo={'linktype_rmi_doors' '0000baa4 (/E-STEER Core/SubSystem Specifications/Application Functions/SF044A HOW)' '#SF044A_82' 'true' 'REQ:SF044A_82' '' } %GIDa_8ee8d4a8_60aa_4acb_915e_eb3a47551d84
  AbsLoFreqTq : Outport  RequirementInfo={'linktype_rmi_doors' '0000baa4 (/E-STEER Core/SubSystem Specifications/Application Functions/SF044A HOW)' '#SF044A_80' 'true' 'REQ:SF044A_80' '' } %GIDa_36abd7fe_7195_4b5e_b140_8896d6280edb  Port=2
  wires:
  Abslt_f32_f32/1 -> Data Store Write1/1, AbsLoFreqTq/1
  FixdToFloat_f32_u16/1 -> Product/1
  VehSpd/1 -> FloatToFixd_u16_f32/1
  HwTq/1 -> FilLpUpdOutp/1
  FilLpUpdOutp3/1 -> Data Store Write6/1, AbsHiFreqTq/1
  FilLpUpdOutp2/1 -> FilHpUpdOutp/1, Abslt_f32_f32/1
  FilHpUpdOutp/1 -> Product/2
  Product/1 -> Abslt_f32_f1/1
  Abslt_f32_f1/1 -> FilLpUpdOutp3/1
  FilLpUpdOutp/1 -> FilLpUpdOutp1/1
  FilLpUpdOutp1/1 -> FilLpUpdOutp2/1
  LnrIntrpn_u16_u16VariXu16VariY/1 -> FixdToFloat_f32_u16/1
  FloatToFixd_u16_f32/1 -> LnrIntrpn_u16_u16VariXu16VariY/1
  Constant/1 -> LnrIntrpn_u16_u16VariXu16VariY/2
  Constant1/1 -> LnrIntrpn_u16_u16VariXu16VariY/3

== system SF044A_HowDetn/HowDetn/HowDetnPer1/Calculate HOW Estimate/CalcEstimn ==
  In1 : Inport
  Action Port : ActionPort  ActionType=then
  CopyRight2 : Subsystem  Description=|  mask(Copyright Information){none=on}
      | Copyright info block.                                               
      |                                                                     
      | Place copyright information at the top of every subsystem in design.
      mask prompts: none "No parameters"
      mask help: Place copyright information at the top of every subsystem in design.
      mask Display:
      | NxtrConf = 'Nexteer Confidential';
      | 
      | sys = bdroot; %handle for the current model ("system")
      | first = get_param(sys,'Created');
      | first = first(end-3:end);  %year is last four digits
      | 
      | last = get_param(sys,'LastModifiedDate');
      | if isempty(last)
      |     last = datestr(now,'yyyy');
      | else
      |     last = last(end-3:end);
      | end
      | 
      | if strcmp(first,last)
      |     fprintf('%s -- Copyright %s Nexteer',NxtrConf,first)
      | else
      |     fprintf('%s -- %s%s- %s Nexteer',NxtrConf,char(169),first,last)
      | end
  Out1 : Outport
  wires:
  In1/1 -> Out1/1

== system SF044A_HowDetn/HowDetn/HowDetnPer1/Calculate HOW Estimate/CopyRight2 ==

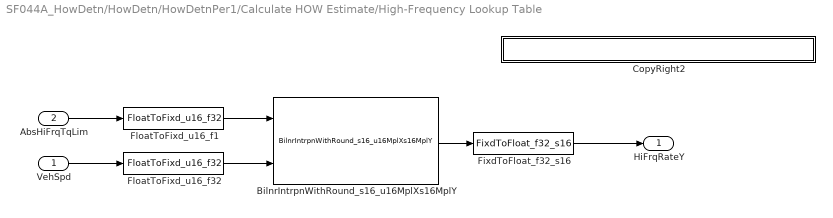
== system SF044A_HowDetn/HowDetn/HowDetnPer1/Calculate HOW Estimate/High-Frequency Lookup Table ==
  VehSpd : Inport
  AbsHiFrqTqLim : Inport  Port=2
  BilnrIntrpnWithRound_s16_u16MplXs16MplY : BilnrIntrpnMplX/BilnrIntrpnWithRound_s16_u16MplXs16MplY  MplXTbl=HowDetnHiFrqRateX  MplYTbl=HowDetnHiFrqRateY  BilnrSelnTbl=HowDetnVehSpd
      settings: AttributesFormatString=Bilnr ( u16MplX , s16MplY )
  CopyRight2 : Subsystem  Description=|  mask(Copyright Information){none=on}
      | Copyright info block.                                               
      |                                                                     
      | Place copyright information at the top of every subsystem in design.
      mask prompts: none "No parameters"
      mask help: Place copyright information at the top of every subsystem in design.
      mask Display:
      | NxtrConf = 'Nexteer Confidential';
      | 
      | sys = bdroot; %handle for the current model ("system")
      | first = get_param(sys,'Created');
      | first = first(end-3:end);  %year is last four digits
      | 
      | last = get_param(sys,'LastModifiedDate');
      | if isempty(last)
      |     last = datestr(now,'yyyy');
      | else
      |     last = last(end-3:end);
      | end
      | 
      | if strcmp(first,last)
      |     fprintf('%s -- Copyright %s Nexteer',NxtrConf,first)
      | else
      |     fprintf('%s -- %s%s- %s Nexteer',NxtrConf,char(169),first,last)
      | end
  FixdToFloat_f32_s16 : FixdToFloat/FixdToFloat_f32_s16  Param1=8
  FloatToFixd_u16_f1 : FloatToFixd/FloatToFixd_u16_f32  Param1=8
  FloatToFixd_u16_f32 : FloatToFixd/FloatToFixd_u16_f32  Param1=7
  HiFrqRateY : Outport
  wires:
  VehSpd/1 -> FloatToFixd_u16_f32/1
  FloatToFixd_u16_f32/1 -> BilnrIntrpnWithRound_s16_u16MplXs16MplY/2
  BilnrIntrpnWithRound_s16_u16MplXs16MplY/1 -> FixdToFloat_f32_s16/1
  AbsHiFrqTqLim/1 -> FloatToFixd_u16_f1/1
  FloatToFixd_u16_f1/1 -> BilnrIntrpnWithRound_s16_u16MplXs16MplY/1
  FixdToFloat_f32_s16/1 -> HiFrqRateY/1

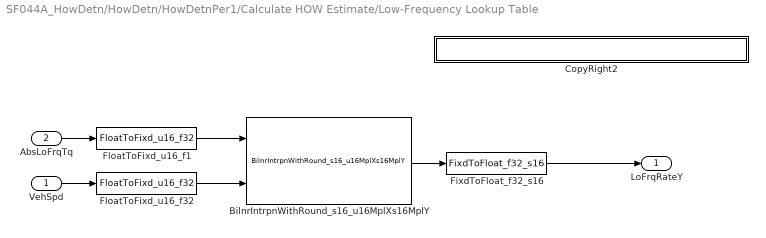
== system SF044A_HowDetn/HowDetn/HowDetnPer1/Calculate HOW Estimate/Low-Frequency Lookup Table ==
  VehSpd : Inport
  AbsLoFrqTq : Inport  Port=2
  BilnrIntrpnWithRound_s16_u16MplXs16MplY : BilnrIntrpnMplX/BilnrIntrpnWithRound_s16_u16MplXs16MplY  MplXTbl=HowDetnLoFrqRateX  MplYTbl=HowDetnLoFrqRateY  BilnrSelnTbl=HowDetnVehSpd
      settings: AttributesFormatString=Bilnr ( u16MplX , s16MplY )
  CopyRight2 : Subsystem  Description=|  mask(Copyright Information){none=on}
      | Copyright info block.                                               
      |                                                                     
      | Place copyright information at the top of every subsystem in design.
      mask prompts: none "No parameters"
      mask help: Place copyright information at the top of every subsystem in design.
      mask Display:
      | NxtrConf = 'Nexteer Confidential';
      | 
      | sys = bdroot; %handle for the current model ("system")
      | first = get_param(sys,'Created');
      | first = first(end-3:end);  %year is last four digits
      | 
      | last = get_param(sys,'LastModifiedDate');
      | if isempty(last)
      |     last = datestr(now,'yyyy');
      | else
      |     last = last(end-3:end);
      | end
      | 
      | if strcmp(first,last)
      |     fprintf('%s -- Copyright %s Nexteer',NxtrConf,first)
      | else
      |     fprintf('%s -- %s%s- %s Nexteer',NxtrConf,char(169),first,last)
      | end
  FixdToFloat_f32_s16 : FixdToFloat/FixdToFloat_f32_s16  Param1=8
  FloatToFixd_u16_f1 : FloatToFixd/FloatToFixd_u16_f32  Param1=8
  FloatToFixd_u16_f32 : FloatToFixd/FloatToFixd_u16_f32  Param1=7
  LoFrqRateY : Outport
  wires:
  FloatToFixd_u16_f32/1 -> BilnrIntrpnWithRound_s16_u16MplXs16MplY/2
  BilnrIntrpnWithRound_s16_u16MplXs16MplY/1 -> FixdToFloat_f32_s16/1
  FloatToFixd_u16_f1/1 -> BilnrIntrpnWithRound_s16_u16MplXs16MplY/1
  VehSpd/1 -> FloatToFixd_u16_f32/1
  AbsLoFrqTq/1 -> FloatToFixd_u16_f1/1
  FixdToFloat_f32_s16/1 -> LoFrqRateY/1

== system SF044A_HowDetn/HowDetn/HowDetnPer1/Calculate HOW Estimate/default ==
  Action Port : ActionPort  ActionType=else
  Constant : Constant  RequirementInfo={} %GIDa_67017ff9_6322_4976_b2c8_c00694960ef8  Value=HOWDETNESTIMNTHD_ULS_F32  OutDataTypeStr=single
  CopyRight2 : Subsystem  Description=|  mask(Copyright Information){none=on}
      | Copyright info block.                                               
      |                                                                     
      | Place copyright information at the top of every subsystem in design.
      mask prompts: none "No parameters"
      mask help: Place copyright information at the top of every subsystem in design.
      mask Display:
      | NxtrConf = 'Nexteer Confidential';
      | 
      | sys = bdroot; %handle for the current model ("system")
      | first = get_param(sys,'Created');
      | first = first(end-3:end);  %year is last four digits
      | 
      | last = get_param(sys,'LastModifiedDate');
      | if isempty(last)
      |     last = datestr(now,'yyyy');
      | else
      |     last = last(end-3:end);
      | end
      | 
      | if strcmp(first,last)
      |     fprintf('%s -- Copyright %s Nexteer',NxtrConf,first)
      | else
      |     fprintf('%s -- %s%s- %s Nexteer',NxtrConf,char(169),first,last)
      | end
  Out : Outport
  wires:
  Constant/1 -> Out/1

== system SF044A_HowDetn/HowDetn/HowDetnPer1/Determine HOW State/CopyRight2 ==

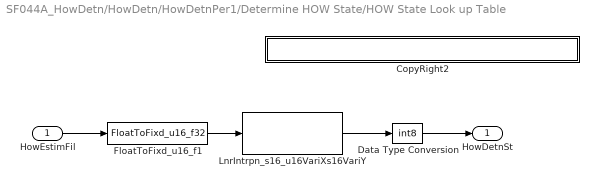
== system SF044A_HowDetn/HowDetn/HowDetnPer1/Determine HOW State/HOW State Look up Table ==
  HowEstimFil : Inport
  CopyRight2 : Subsystem  Description=|  mask(Copyright Information){none=on}
      | Copyright info block.                                               
      |                                                                     
      | Place copyright information at the top of every subsystem in design.
      mask prompts: none "No parameters"
      mask help: Place copyright information at the top of every subsystem in design.
      mask Display:
      | NxtrConf = 'Nexteer Confidential';
      | 
      | sys = bdroot; %handle for the current model ("system")
      | first = get_param(sys,'Created');
      | first = first(end-3:end);  %year is last four digits
      | 
      | last = get_param(sys,'LastModifiedDate');
      | if isempty(last)
      |     last = datestr(now,'yyyy');
      | else
      |     last = last(end-3:end);
      | end
      | 
      | if strcmp(first,last)
      |     fprintf('%s -- Copyright %s Nexteer',NxtrConf,first)
      | else
      |     fprintf('%s -- %s%s- %s Nexteer',NxtrConf,char(169),first,last)
      | end
  Data Type Conversion : DataTypeConversion  OutDataTypeStr=int8
  FloatToFixd_u16_f1 : FloatToFixd/FloatToFixd_u16_f32  Param1=8
  LnrIntrpn_s16_u16VariXs16VariY : LnrIntrpn/LnrIntrpn_s16_u16VariXs16VariY  RequirementInfo={} %GIDa_1ceff8d9_cb44_435a_8fb8_bb742ada6bbe  XTbl=HowDetnStThdX  YTbl=HOWSTY_CNT_S15P0
      settings: AttributesFormatString=Lnr ( u16VariX , s16VariY )
  HowDetnSt : Outport
  wires:
  HowEstimFil/1 -> FloatToFixd_u16_f1/1
  FloatToFixd_u16_f1/1 -> LnrIntrpn_s16_u16VariXs16VariY/1
  LnrIntrpn_s16_u16VariXs16VariY/1 -> Data Type Conversion/1
  Data Type Conversion/1 -> HowDetnSt/1

== system SF044A_HowDetn/HowDetn/HowDetnPer1/Determine HOW State/Pass ==
  Input : Inport
  Action Port : ActionPort  ActionType=then
  CopyRight2 : Subsystem  Description=|  mask(Copyright Information){none=on}
      | Copyright info block.                                               
      |                                                                     
      | Place copyright information at the top of every subsystem in design.
      mask prompts: none "No parameters"
      mask help: Place copyright information at the top of every subsystem in design.
      mask Display:
      | NxtrConf = 'Nexteer Confidential';
      | 
      | sys = bdroot; %handle for the current model ("system")
      | first = get_param(sys,'Created');
      | first = first(end-3:end);  %year is last four digits
      | 
      | last = get_param(sys,'LastModifiedDate');
      | if isempty(last)
      |     last = datestr(now,'yyyy');
      | else
      |     last = last(end-3:end);
      | end
      | 
      | if strcmp(first,last)
      |     fprintf('%s -- Copyright %s Nexteer',NxtrConf,first)
      | else
      |     fprintf('%s -- %s%s- %s Nexteer',NxtrConf,char(169),first,last)
      | end
  HowDetnSt : Outport
  wires:
  Input/1 -> HowDetnSt/1

== system SF044A_HowDetn/HowDetn/HowDetnPer1/Determine HOW State/Zero ==
  Action Port : ActionPort  ActionType=else
  Constant : Constant  Value=0  OutDataTypeStr=int8
      settings: AttributesFormatString=%<OutDataTypeStr>
  CopyRight2 : Subsystem  Description=|  mask(Copyright Information){none=on}
      | Copyright info block.                                               
      |                                                                     
      | Place copyright information at the top of every subsystem in design.
      mask prompts: none "No parameters"
      mask help: Place copyright information at the top of every subsystem in design.
      mask Display:
      | NxtrConf = 'Nexteer Confidential';
      | 
      | sys = bdroot; %handle for the current model ("system")
      | first = get_param(sys,'Created');
      | first = first(end-3:end);  %year is last four digits
      | 
      | last = get_param(sys,'LastModifiedDate');
      | if isempty(last)
      |     last = datestr(now,'yyyy');
      | else
      |     last = last(end-3:end);
      | end
      | 
      | if strcmp(first,last)
      |     fprintf('%s -- Copyright %s Nexteer',NxtrConf,first)
      | else
      |     fprintf('%s -- %s%s- %s Nexteer',NxtrConf,char(169),first,last)
      | end
  HowDetnSt : Outport
  wires:
  Constant/1 -> HowDetnSt/1

== system SF044A_HowDetn/HowDetn/HowDetnPer1/Filter HwTq/CopyRight2 ==

== system SF044A_HowDetn/HowDetn/HowDetnPer1/Calculate HOW Estimate/CalcEstimn/CopyRight2 ==

== system SF044A_HowDetn/HowDetn/HowDetnPer1/Calculate HOW Estimate/High-Frequency Lookup Table/CopyRight2 ==
